simulink model "SerialSendReceive"  (R2020b)
settings: Solver=FixedStepDiscrete  StartTime=0.0  StopTime=inf  FixedStep=0.01  RelTol=1e-3
libraries: arduinolib x16, simulink x2, aerolibanimutils x1, commutil2 x1
settings Model: SimulationMode=external  ExtModeTrigDuration=2  Creator=Pablo  LastModifiedBy=Pablo
settings SolverCC: AutoInsertRateTranBlk=on
settings DataIOCC: ReturnWorkspaceOutputs=off
settings OptimizationCC: PassReuseOutputArgsAs=Individual arguments  MaxStackSize=64  EfficientTunableParamExpr=on
settings DebuggingCC: ParameterOverflowMsg=none  ParameterTunabilityLossMsg=error  ArithmeticOperatorsInVariantConditions=warning
settings HardwareCC: ProdBitPerInt=16  ProdBitPerPointer=16  ProdBitPerSizeT=16  ProdBitPerPtrDiffT=16  ProdLargestAtomicFloat=None  ProdWordSize=8  ProdHWDeviceType=Atmel->AVR  UseEmbeddedCoderFeatures=off  UseSimulinkCoderFeatures=off
settings SFSimCC: SimUseLocalCustomCode=off  MATLABDynamicMemAlloc=off  CustomCodeUndefinedFunction=UseInterfaceOnly
settings RTWCC: Description=Embedded Coder  SystemTargetFile=ert.tlc  HardwareBoard=Arduino Mega 2560  TemplateMakefile=ert_default_tmf  GenerateReport=on  RTWUseLocalCustomCode=off  Toolchain=Arduino AVR  BuildConfiguration=Faster Runs  IncludeHyperlinkInReport=on  LaunchReport=on  GenerateTraceInfo=on  GenerateTraceReport=on  GenerateTraceReportSl=on  GenerateTraceReportSf=on  GenerateTraceReportEml=on
settings CodeAppCC: ForceParamTrailComments=on  IgnoreCustomStorageClasses=off  OperatorAnnotations=on  SimulinkDataObjDesc=on  SFDataObjDesc=on  InsertBlockDesc=on
settings ERTTargetCC: SupportContinuousTime=on  SupportNonInlinedSFcns=on  SupportVariableSizeSignals=on

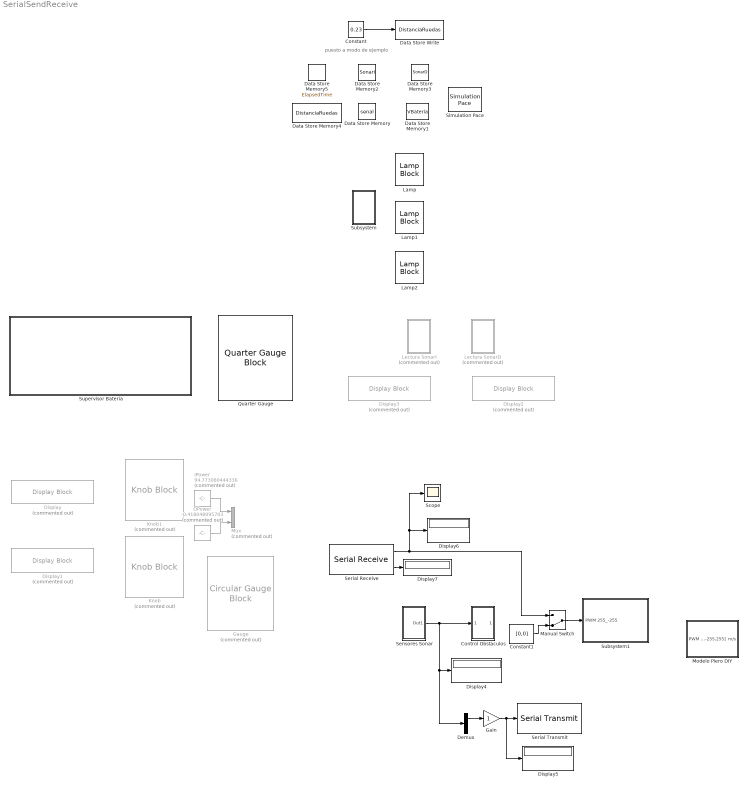
== system SerialSendReceive ==
  note: puesto a modo de ejemplo
  Constant : Constant  Value=0.23
  Constant1 : Constant  Value=[0,0]
  Control Obstaculos : Subsystem
  DPower : Constant  Commented=on  Value=-0.418048095703  OutDataTypeStr=int16
  Data Store Memory : DataStoreMemory  DataStoreName=senal  ReadBeforeWriteMsg=warning  WriteAfterWriteMsg=warning  WriteAfterReadMsg=warning  ShowAdditionalParam=off  OutDataTypeStr=uint8
  Data Store Memory1 : DataStoreMemory  DataStoreName=VBateria  ReadBeforeWriteMsg=warning  WriteAfterWriteMsg=warning  WriteAfterReadMsg=warning  ShowAdditionalParam=off  OutDataTypeStr=double
  Data Store Memory2 : DataStoreMemory  DataStoreName=SonarI  ReadBeforeWriteMsg=warning  WriteAfterWriteMsg=warning  WriteAfterReadMsg=warning  ShowAdditionalParam=off  OutDataTypeStr=uint8
  Data Store Memory3 : DataStoreMemory  DataStoreName=SonarD  ReadBeforeWriteMsg=warning  WriteAfterWriteMsg=warning  WriteAfterReadMsg=warning  ShowAdditionalParam=off  OutDataTypeStr=uint8
  Data Store Memory4 : DataStoreMemory  DataStoreName=DistanciaRuedas  ReadBeforeWriteMsg=warning  WriteAfterWriteMsg=warning  WriteAfterReadMsg=warning  ShowAdditionalParam=off  OutDataTypeStr=double
  Data Store Memory5 : DataStoreMemory  DataStoreName=ElapsedTime  ReadBeforeWriteMsg=warning  WriteAfterWriteMsg=warning  WriteAfterReadMsg=warning  ShowAdditionalParam=off
  Data Store Write : DataStoreWrite  DataStoreName=DistanciaRuedas
  Demux : Demux  Outputs=2
  Display{,1..3} (4 alike) : DisplayBlock  Commented=on  LabelPosition=Hide
  Display{4..7} (4 alike) : Display
  Gain : Gain  OutDataTypeStr=uint8
  Gauge : CircularGaugeBlock  Commented=on  ScaleMax=255
  IPower : Constant  Commented=on  Value=94.773080444336  OutDataTypeStr=int16
  Knob : KnobBlock  Commented=on
  Knob1 : KnobBlock  Commented=on
  Lamp : LampBlock
  Lamp1 : LampBlock
  Lamp2 : LampBlock
  Lectura SonarD : Subsystem  Commented=on
  Lectura SonarI : Subsystem  Commented=on
  Manual Switch : ManualSwitch  CurrentSetting=0
  Modelo Piero DIY : Subsystem
  Mux : Mux  Commented=on  Inputs=2
  Quarter Gauge : QuarterGaugeBlock  ScaleMin=10  ScaleMax=13
  Scope : Scope
  Sensores Sonar : Subsystem
  Serial Receive : arduinolib/Serial Receive  isARMArch=off  portNumber=3  DataType=uint8  Datalength=2  SampleTime=0.1  showOutStatus=on  blockPlatform=arduino
      settings: SourceProductBaseCode=ARDUINO
  Serial Transmit : arduinolib/Serial Transmit  portNumber=3  sendmode=write  sendformat=Decimal  floatprecision=2  blockPlatform=arduino
  Simulation Pace : aerolibanimutils/Simulation Pace  SimulationPace=1  SleepMode=MATLAB Thread  OutputPaceError=off  SampleTime=-1
  Subsystem : Subsystem
  Subsystem1 : Subsystem
  Supervisor Bateria : Subsystem
  wires:
  IPower/1 -> Mux/1
  DPower/1 -> Mux/2
  Constant/1 -> Data Store Write/1
  Sensores Sonar/1(Out1) -> Demux/1, Display4/1, Control Obstaculos/1(In1)
  Serial Receive/1 -> Scope/1, Display6/1, Manual Switch/1
  Serial Receive/2 -> Display7/1
  Manual Switch/1 -> Subsystem1/1(PWM 255_-255)
  Constant1/1 -> Manual Switch/2
  Demux/1 -> Gain/1
  Gain/1 -> Display5/1, Serial Transmit/1

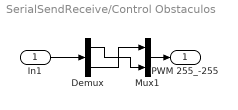
== system SerialSendReceive/Control Obstaculos ==
  In1 : Inport
  Demux : Demux  Outputs=2
  Mux1 : Mux  Inputs=2
  PWM 255_-255 : Outport  VectorParamsAs1DForOutWhenUnconnected=off
  wires:
  Mux1/1 -> PWM 255_-255/1
  Demux/2 -> Mux1/1
  Demux/1 -> Mux1/2
  In1/1 -> Demux/1

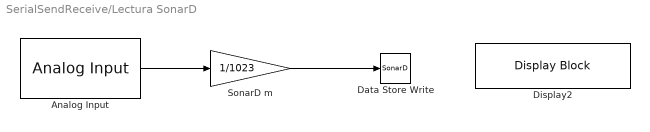
== system SerialSendReceive/Lectura SonarD ==
  Analog Input : arduinolib/Analog Input  pinNumber=2  sampleTime=1  blockPlatform=arduino
  Data Store Write : DataStoreWrite  DataStoreName=SonarD
  Display2 : DisplayBlock  LabelPosition=Hide
  SonarD m : Gain  Gain=1/1023  ParamDataTypeStr=uint8  OutDataTypeStr=uint8
  wires:
  Analog Input/1 -> SonarD m/1
  SonarD m/1 -> Data Store Write/1

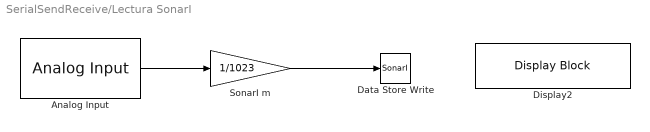
== system SerialSendReceive/Lectura SonarI ==
  Analog Input : arduinolib/Analog Input  pinNumber=1  sampleTime=1  blockPlatform=arduino
  Data Store Write : DataStoreWrite  DataStoreName=SonarI
  Display2 : DisplayBlock  LabelPosition=Hide
  SonarI m : Gain  Gain=1/1023  ParamDataTypeStr=uint8  OutDataTypeStr=uint8
  wires:
  Analog Input/1 -> SonarI m/1
  SonarI m/1 -> Data Store Write/1

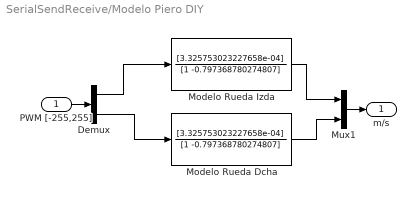
== system SerialSendReceive/Modelo Piero DIY ==
  PWM [-255,255] : Inport
  Demux : Demux  Outputs=2
  Modelo Rueda Dcha : DiscreteFilter  Numerator=[3.325753023227658e-04]  Denominator=[1 -0.797368780274807]
  Modelo Rueda Izda : DiscreteFilter  Numerator=[3.325753023227658e-04]  Denominator=[1 -0.797368780274807]
  Mux1 : Mux  Inputs=2
  m/s : Outport  VectorParamsAs1DForOutWhenUnconnected=off
  wires:
  PWM [-255,255]/1 -> Demux/1
  Mux1/1 -> m/s/1
  Modelo Rueda Izda/1 -> Mux1/1
  Demux/1 -> Modelo Rueda Izda/1
  Modelo Rueda Dcha/1 -> Mux1/2
  Demux/2 -> Modelo Rueda Dcha/1

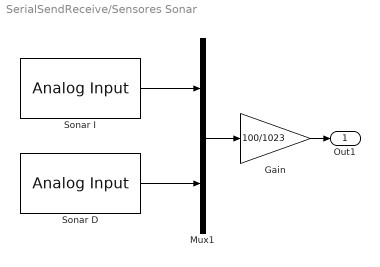
== system SerialSendReceive/Sensores Sonar ==
  Gain : Gain  Gain=100/1023
  Mux1 : Mux  Inputs=2
  Sonar D : arduinolib/Analog Input  pinNumber=1  ReadResultsOnly=off  ConversionTriggerSource=Software  ExternalTriggerType=uint32( 0 )  OutputDataType=uint16  EnableConversionCompleteNotify=off  EnableOuputStatus=off  SampleTime=0.1  blockPlatform=arduino
  Sonar I : arduinolib/Analog Input  pinNumber=0  ReadResultsOnly=off  ConversionTriggerSource=Software  ExternalTriggerType=uint32( 0 )  OutputDataType=uint16  EnableConversionCompleteNotify=off  EnableOuputStatus=off  SampleTime=0.1  blockPlatform=arduino
  Out1 : Outport  VectorParamsAs1DForOutWhenUnconnected=off
  wires:
  Gain/1 -> Out1/1
  Mux1/1 -> Gain/1
  Sonar I/1 -> Mux1/1
  Sonar D/1 -> Mux1/2

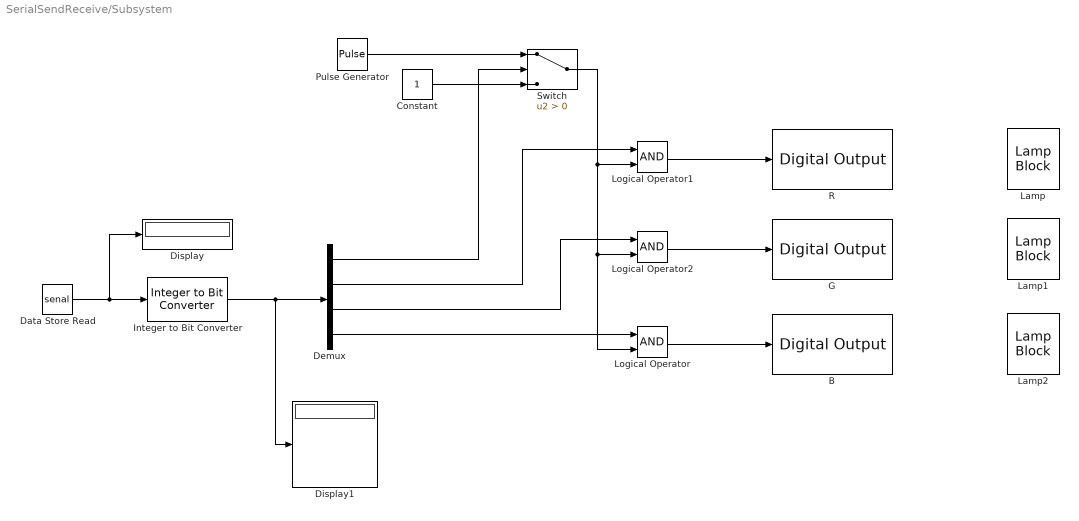
== system SerialSendReceive/Subsystem ==
  B : arduinolib/Digital Output  pinNumber=49  Direction=output  blockPlatform=arduino
  Constant : Constant
  Data Store Read : DataStoreRead  DataStoreName=senal
  Demux : Demux
  Display : Display
  Display1 : Display
  G : arduinolib/Digital Output  pinNumber=53  Direction=output  blockPlatform=arduino
  Integer to Bit Converter : commutil2/Integer to Bit Converter  nbits=4  signedInputValues=Unsigned  bitOrder=MSB first  outDtype=Inherit via internal rule
  Lamp : LampBlock
  Lamp1 : LampBlock
  Lamp2 : LampBlock
  Logical Operator : Logic  AllPortsSameDT=off  OutDataTypeStr=boolean
  Logical Operator1 : Logic  AllPortsSameDT=off  OutDataTypeStr=boolean
  Logical Operator2 : Logic  AllPortsSameDT=off  OutDataTypeStr=boolean
  Pulse Generator : DiscretePulseGenerator  PulseType=Time based  Period=1  PulseWidth=50
  R : arduinolib/Digital Output  pinNumber=51  Direction=output  blockPlatform=arduino
  Switch : Switch  Criteria=u2 > Threshold
  wires:
  Switch/1 -> Logical Operator/2, Logical Operator2/2, Logical Operator1/2
  Pulse Generator/1 -> Switch/1
  Demux/1 -> Switch/2
  Logical Operator/1 -> B/1
  Logical Operator1/1 -> R/1
  Logical Operator2/1 -> G/1
  Demux/4 -> Logical Operator/1
  Demux/3 -> Logical Operator2/1
  Demux/2 -> Logical Operator1/1
  Constant/1 -> Switch/3
  Integer to Bit Converter/1 -> Display1/1, Demux/1
  Data Store Read/1 -> Display/1, Integer to Bit Converter/1

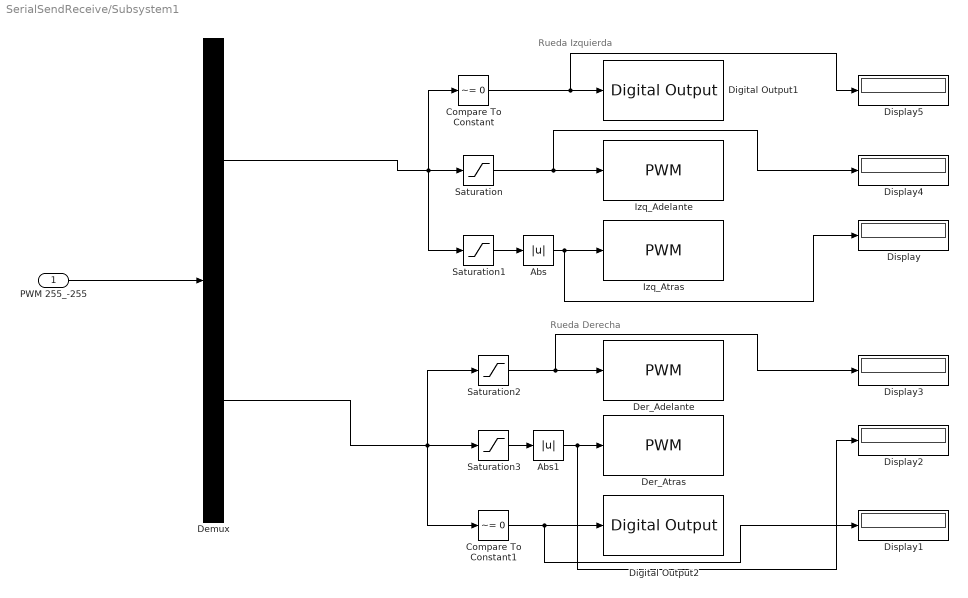
== system SerialSendReceive/Subsystem1 ==
  note: Rueda Derecha
  note: Rueda Izquierda
  PWM 255_-255 : Inport
  Abs : Abs  OutDataTypeStr=uint8
  Abs1 : Abs  OutDataTypeStr=uint8
  Compare To Constant : simulink/Logic and Bit Operations/Compare To Constant  relop=~=  const=0  OutDataTypeStr=boolean
  Compare To Constant1 : simulink/Logic and Bit Operations/Compare To Constant  relop=~=  const=0  OutDataTypeStr=boolean
  Demux : Demux  Outputs=2
  Der_Adelante : arduinolib/PWM  pinNumber=8  frequencyType=Default  desiredFrequency=490.2  achievableFrequency=490.2
  Der_Atras : arduinolib/PWM  pinNumber=9  frequencyType=Default  desiredFrequency=490.2  achievableFrequency=490.2
  Digital Output1 : arduinolib/Digital Output  pinNumber=5  Direction=output  blockPlatform=arduino
  Digital Output2 : arduinolib/Digital Output  pinNumber=10  Direction=output  blockPlatform=arduino
  Display{,1..5} (6 alike) : Display
  Izq_Adelante : arduinolib/PWM  pinNumber=6  frequencyType=Default  desiredFrequency=490.2  achievableFrequency=490.2
  Izq_Atras : arduinolib/PWM  pinNumber=7  frequencyType=Default  desiredFrequency=490.2  achievableFrequency=490.2
  Saturation : Saturate  UpperLimit=255  LowerLimit=0
  Saturation1 : Saturate  UpperLimit=0  LowerLimit=-255  OutDataTypeStr=uint16
  Saturation2 : Saturate  UpperLimit=255  LowerLimit=0
  Saturation3 : Saturate  UpperLimit=0  LowerLimit=-255
  wires:
  Saturation/1 -> Display4/1, Izq_Adelante/1
  Compare To Constant/1 -> Display5/1, Digital Output1/1
  Saturation1/1 -> Abs/1
  PWM 255_-255/1 -> Demux/1
  Demux/1 -> Saturation1/1, Compare To Constant/1, Saturation/1
  Abs/1 -> Display/1, Izq_Atras/1
  Saturation3/1 -> Abs1/1
  Demux/2 -> Compare To Constant1/1, Saturation2/1, Saturation3/1
  Compare To Constant1/1 -> Display1/1, Digital Output2/1
  Abs1/1 -> Display2/1, Der_Atras/1
  Saturation2/1 -> Display3/1, Der_Adelante/1

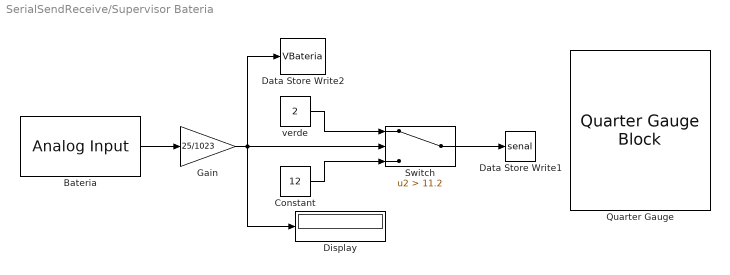
== system SerialSendReceive/Supervisor Bateria ==
  "Bateria " : arduinolib/Analog Input  pinNumber=2  ReadResultsOnly=off  ConversionTriggerSource=Software  ExternalTriggerType=uint32( 0 )  OutputDataType=uint16  EnableConversionCompleteNotify=off  EnableOuputStatus=off  SampleTime=1  blockPlatform=arduino
  Constant : Constant  Value=12
  Data Store Write1 : DataStoreWrite  DataStoreName=senal
  Data Store Write2 : DataStoreWrite  DataStoreName=VBateria
  Display : Display
  Gain : Gain  Gain=25/1023  OutDataTypeStr=double
  Quarter Gauge : QuarterGaugeBlock  ScaleMin=10  ScaleMax=13
  Switch : Switch  Criteria=u2 > Threshold  Threshold=11.2  OutDataTypeStr=uint8
  verde : Constant  Value=2
  wires:
  "Bateria "/1 -> Gain/1
  Constant/1 -> Switch/3
  Gain/1 -> Switch/2, Display/1, Data Store Write2/1
  verde/1 -> Switch/1
  Switch/1 -> Data Store Write1/1
